simulink subsystem "Linear2DimensionCarModel"  (R2022b)
settings: Solver=VariableStepAuto  StartTime=0.0  StopTime=10.0  RelTol=1e-3
settings Model: Creator=ASOAT  LastModifiedBy=ASOAT

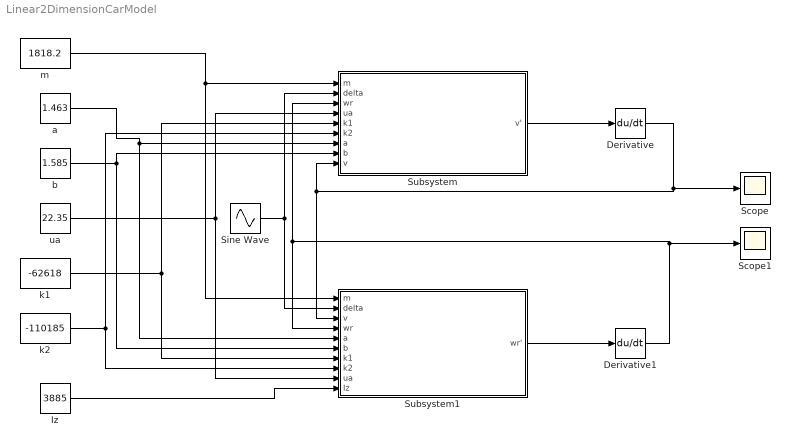
== system Linear2DimensionCarModel ==
  Derivative : Derivative
  Derivative1 : Derivative
  Iz : Constant  Value=3885
  Scope : Scope
  Scope1 : Scope
  Sine Wave : Sin  Amplitude=3.14/2  SampleTime=0
  Subsystem : Subsystem
  Subsystem1 : Subsystem
  a : Constant  Value=1.463
  b : Constant  Value=1.585
  k1 : Constant  Value=-62618
  k2 : Constant  Value=-110185
  m : Constant  Value=1818.2
  ua : Constant  Value=22.35
  wires:
  ua/1 -> Subsystem/4(ua), Subsystem1/9(ua)
  k1/1 -> Subsystem/5(k1), Subsystem1/7(k1)
  k2/1 -> Subsystem1/8(k2), Subsystem/6(k2)
  Subsystem/1(v') -> Derivative/1
  Derivative/1 -> Subsystem/9(v), Subsystem1/3(v), Scope/1
  Subsystem1/1(wr') -> Derivative1/1
  Derivative1/1 -> Subsystem/3(wr), Subsystem1/4(wr), Scope1/1
  a/1 -> Subsystem1/5(a), Subsystem/7(a)
  b/1 -> Subsystem1/6(b), Subsystem/8(b)
  Sine Wave/1 -> Subsystem1/2(delta), Subsystem/2(delta)
  m/1 -> Subsystem1/1(m), Subsystem/1(m)
  Iz/1 -> Subsystem1/10(Iz)

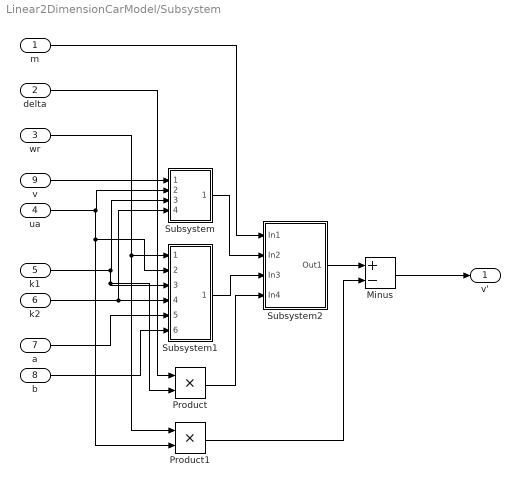
== system Linear2DimensionCarModel/Subsystem ==
  m : Inport
  delta : Inport  Port=2
  wr : Inport  Port=3
  ua : Inport  Port=4
  k1 : Inport  Port=5
  k2 : Inport  Port=6
  a : Inport  Port=7
  b : Inport  Port=8
  v : Inport  Port=9
  Minus : Sum  Inputs=+-
  Product : Product
  Product1 : Product
  Subsystem : Subsystem
  Subsystem1 : Subsystem
  Subsystem2 : Subsystem
  v' : Outport
  wires:
  v/1 -> Subsystem/1(In1)
  ua/1 -> Product1/2, Subsystem1/2(In2), Subsystem/2(In2)
  k1/1 -> Product/2, Subsystem1/3(In3), Subsystem/3(In3)
  k2/1 -> Subsystem1/4(In4), Subsystem/4(In4)
  wr/1 -> Product1/1, Subsystem1/1(In1)
  a/1 -> Subsystem1/5(In5)
  b/1 -> Subsystem1/6(In6)
  delta/1 -> Product/1
  m/1 -> Subsystem2/1(In1)
  Subsystem/1(Out1) -> Subsystem2/2(In2)
  Subsystem1/1(Out1) -> Subsystem2/3(In3)
  Product/1 -> Subsystem2/4(In4)
  Subsystem2/1(Out1) -> Minus/1
  Product1/1 -> Minus/2
  Minus/1 -> v'/1

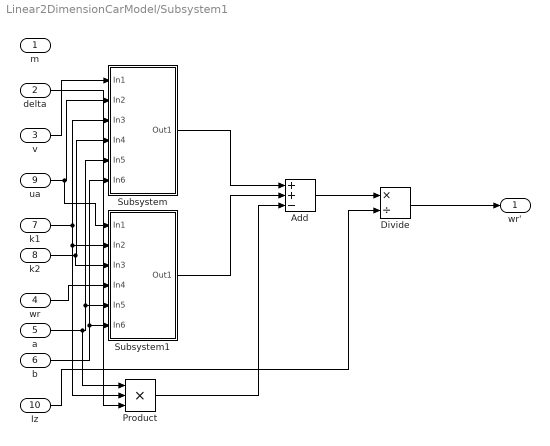
== system Linear2DimensionCarModel/Subsystem1 ==
  m : Inport
  delta : Inport  Port=2
  v : Inport  Port=3
  wr : Inport  Port=4
  a : Inport  Port=5
  b : Inport  Port=6
  k1 : Inport  Port=7
  k2 : Inport  Port=8
  ua : Inport  Port=9
  Iz : Inport  Port=10
  Add : Sum  Inputs=++-
  Divide : Product  Inputs=*/
  Product : Product  Inputs=3
  Subsystem : Subsystem
  Subsystem1 : Subsystem
  wr' : Outport
  wires:
  v/1 -> Subsystem/1(In1)
  ua/1 -> Subsystem1/1(In1), Subsystem/2(In2)
  k1/1 -> Product/2, Subsystem1/2(In2), Subsystem/3(In3)
  k2/1 -> Subsystem1/3(In3), Subsystem/4(In4)
  a/1 -> Product/1, Subsystem1/5(In5), Subsystem/5(In5)
  b/1 -> Subsystem1/6(In6), Subsystem/6(In6)
  wr/1 -> Subsystem1/4(In4)
  delta/1 -> Product/3
  Subsystem/1(Out1) -> Add/1
  Subsystem1/1(Out1) -> Add/2
  Product/1 -> Add/3
  Add/1 -> Divide/1
  Iz/1 -> Divide/2
  Divide/1 -> wr'/1

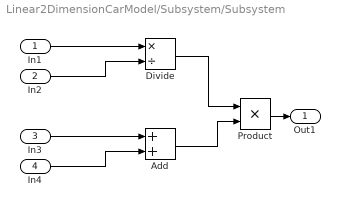
== system Linear2DimensionCarModel/Subsystem/Subsystem ==
  In1 : Inport
  In2 : Inport  Port=2
  In3 : Inport  Port=3
  In4 : Inport  Port=4
  Add : Sum
  Divide : Product  Inputs=*/
  Product : Product
  Out1 : Outport
  wires:
  Divide/1 -> Product/1
  Add/1 -> Product/2
  In3/1 -> Add/1
  In4/1 -> Add/2
  In2/1 -> Divide/2
  In1/1 -> Divide/1
  Product/1 -> Out1/1

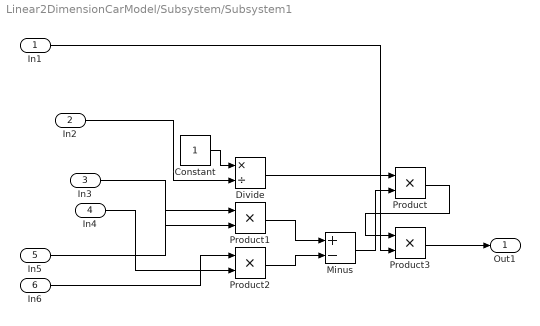
== system Linear2DimensionCarModel/Subsystem/Subsystem1 ==
  In1 : Inport
  In2 : Inport  Port=2
  In3 : Inport  Port=3
  In4 : Inport  Port=4
  In5 : Inport  Port=5
  In6 : Inport  Port=6
  Constant : Constant
  Divide : Product  Inputs=*/
  Minus : Sum  Inputs=+-
  Product{,1..3} (4 alike) : Product
  Out1 : Outport
  wires:
  Constant/1 -> Divide/1
  Minus/1 -> Product/2
  In3/1 -> Product1/2
  Product3/1 -> Out1/1
  In4/1 -> Product2/2
  Product/1 -> Product3/1
  Divide/1 -> Product/1
  Product2/1 -> Minus/2
  In1/1 -> Product3/2
  Product1/1 -> Minus/1
  In6/1 -> Product2/1
  In5/1 -> Product1/1
  In2/1 -> Divide/2

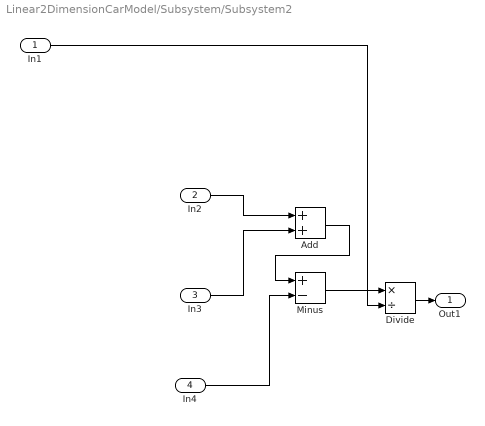
== system Linear2DimensionCarModel/Subsystem/Subsystem2 ==
  In1 : Inport
  In2 : Inport  Port=2
  In3 : Inport  Port=3
  In4 : Inport  Port=4
  Add : Sum
  Divide : Product  Inputs=*/
  Minus : Sum  Inputs=+-
  Out1 : Outport
  wires:
  Divide/1 -> Out1/1
  Add/1 -> Minus/1
  In2/1 -> Add/1
  Minus/1 -> Divide/1
  In4/1 -> Minus/2
  In3/1 -> Add/2
  In1/1 -> Divide/2

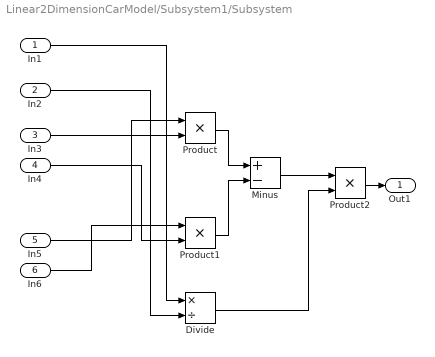
== system Linear2DimensionCarModel/Subsystem1/Subsystem ==
  In1 : Inport
  In2 : Inport  Port=2
  In3 : Inport  Port=3
  In4 : Inport  Port=4
  In5 : Inport  Port=5
  In6 : Inport  Port=6
  Divide : Product  Inputs=*/
  Minus : Sum  Inputs=+-
  Product : Product
  Product1 : Product
  Product2 : Product
  Out1 : Outport
  wires:
  In2/1 -> Divide/2
  Minus/1 -> Product2/1
  Product1/1 -> Minus/2
  Product/1 -> Minus/1
  Product2/1 -> Out1/1
  Divide/1 -> Product2/2
  In6/1 -> Product1/1
  In5/1 -> Product/1
  In1/1 -> Divide/1
  In4/1 -> Product1/2
  In3/1 -> Product/2

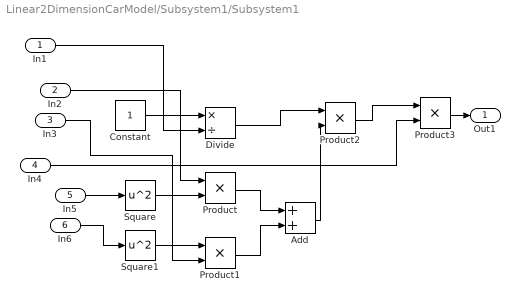
== system Linear2DimensionCarModel/Subsystem1/Subsystem1 ==
  In1 : Inport
  In2 : Inport  Port=2
  In3 : Inport  Port=3
  In4 : Inport  Port=4
  In5 : Inport  Port=5
  In6 : Inport  Port=6
  Add : Sum
  Constant : Constant
  Divide : Product  Inputs=*/
  Product{,1..3} (4 alike) : Product
  Square : Math  Operator=square
  Square1 : Math  Operator=square
  Out1 : Outport
  wires:
  Product2/1 -> Product3/1
  In1/1 -> Divide/2
  Divide/1 -> Product2/1
  Square1/1 -> Product1/1
  Add/1 -> Product2/2
  In3/1 -> Product1/2
  Square/1 -> Product/2
  Constant/1 -> Divide/1
  Product/1 -> Add/1
  Product1/1 -> Add/2
  In5/1 -> Square/1
  In2/1 -> Product/1
  Product3/1 -> Out1/1
  In6/1 -> Square1/1
  In4/1 -> Product3/2
